simulink model "Pokus07_Display"  (Simulink 8.1)
settings: Solver=ode45  StartTime=0.0  StopTime=10.0  RelTol=1e-3
undefined symbols (not defined in the file): A, ARROW_DOWN, ARROW_LEFT, ARROW_RIGHT, ARROW_UP, ASTERISK, B, BACKSLASH, C, COLON, COMMA, CROSS, CURSOR, D, DOT, ending_column_index, ending_row_index, EQUAL, EXCLAMATION_MARK, F, framebuffer, G, GREATER_THAN, H, HEIGHT, hot, I, J, K, L, LEFT_PARENTHESES, LESS_THAN, M, MINUS, N, O, P, PERCENT, PLUS, POS_X, POS_Y, Q, QUESTION_MARK, QUOTE, R, RECTANGLE, RIGHT_PARENTHESES, S, SEMICOLON, SHARP, SLASH, SPACE, starting_column_index, starting_row_index, T, U, UNDERSCORE, V, W, WIDTH ... (+6)
libraries: dspmtrx3 x197, Common_Library x69, commutil2 x53, simulink_extras x1, dspsnks4 x1
(part 1 of 6)
settings Model: Creator=uzivatel  LastModifiedBy=uzivatel
settings DataIOCC: SignalLoggingSaveFormat=Dataset
settings OptimizationCC: ExpressionDepthLimit=128
settings DebuggingCC: FcnCallInpInsideContextMsg=EnableAllAsError
settings GRTTargetCC: CombineOutputUpdateFcns=on  GRTInterface=off

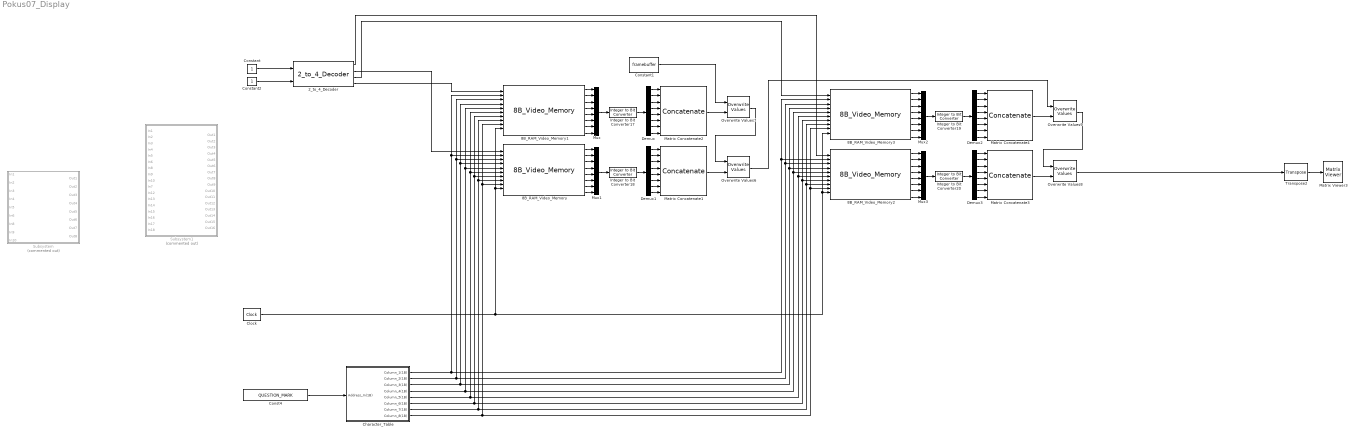
== system Pokus07_Display ==
  2_to_4_Decoder : Common_Library/Decoders/2_to_4_Decoder
  8B_RAM_Video_Memory{,1..3} (4 alike) : Common_Library/Memory_Blocks/8B_Video_Memory
  Character_Table : Subsystem
  Clock : simulink_extras/Flip Flops/Clock  period=1
  Const4 : Constant  Value=QUESTION_MARK  OutDataTypeStr=uint8
  Constant : Constant  OutDataTypeStr=boolean
  Constant1 : Constant  Value=framebuffer  OutDataTypeStr=uint8
  Constant2 : Constant  OutDataTypeStr=boolean
  Demux{,1..3} (4 alike) : Demux  Outputs=8
  Integer to Bit Converter{17..20} (4 alike) : commutil2/Integer to Bit Converter  nbits=8  signedInputValues=Unsigned  bitOrder=MSB first  outDtype=uint8
  Matrix Concatenate{1..4} (4 alike) : Concatenate  NumInputs=8  Mode=Multidimensional array  ConcatenateDimension=2
  Matrix Viewer3 : dspsnks4/Matrix Viewer  ImageParams=off  CMapStr=hot(256)  AxisColorbar=on  AxisParams=off  AxisOrigin=Upper left corner  XLabel=X-axis  YLabel=Y-axis  ZLabel=Z-axis  FigPos=[POS_X POS_Y-140 WIDTH HEIGHT]  AxisZoom=on
      settings: YMin=0  YMax=1.0
  Mux{,1..3} (4 alike) : Mux  Inputs=8
  Overwrite Values6 : dspmtrx3/Overwrite Values  OverWriteDiag=Submatrix  valFrom2ndIP=Second input port  ConstValue=0  RowSpan=Range of rows  RowStartMode=Index  RowStartIndex=starting_row_index(2)  RowEndMode=Index  RowEndIndex=ending_row_index(2)  ColSpan=Range of columns  ColStartMode=Index  ColStartIndex=starting_column_index(1)  ColEndMode=Index  ColEndIndex=ending_column_index(1)  DiagSpan=Range of elements  DiagStartMode=Index  DiagStartIndex=2  DiagEndMode=Index  DiagEndIndex=4
  Overwrite Values7 : dspmtrx3/Overwrite Values  OverWriteDiag=Submatrix  valFrom2ndIP=Second input port  ConstValue=0  RowSpan=Range of rows  RowStartMode=Index  RowStartIndex=starting_row_index(1)  RowEndMode=Index  RowEndIndex=ending_row_index(1)  ColSpan=Range of columns  ColStartMode=Index  ColStartIndex=starting_column_index(1)  ColEndMode=Index  ColEndIndex=ending_column_index(1)  DiagSpan=Range of elements  DiagStartMode=Index  DiagStartIndex=2  DiagEndMode=Index  DiagEndIndex=4
  Overwrite Values8 : dspmtrx3/Overwrite Values  OverWriteDiag=Submatrix  valFrom2ndIP=Second input port  ConstValue=0  RowSpan=Range of rows  RowStartMode=Index  RowStartIndex=starting_row_index(2)  RowEndMode=Index  RowEndIndex=ending_row_index(2)  ColSpan=Range of columns  ColStartMode=Index  ColStartIndex=starting_column_index(2)  ColEndMode=Index  ColEndIndex=ending_column_index(2)  DiagSpan=Range of elements  DiagStartMode=Index  DiagStartIndex=2  DiagEndMode=Index  DiagEndIndex=4
  Overwrite Values9 : dspmtrx3/Overwrite Values  OverWriteDiag=Submatrix  valFrom2ndIP=Second input port  ConstValue=0  RowSpan=Range of rows  RowStartMode=Index  RowStartIndex=starting_row_index(1)  RowEndMode=Index  RowEndIndex=ending_row_index(1)  ColSpan=Range of columns  ColStartMode=Index  ColStartIndex=starting_column_index(2)  ColEndMode=Index  ColEndIndex=ending_column_index(2)  DiagSpan=Range of elements  DiagStartMode=Index  DiagStartIndex=2  DiagEndMode=Index  DiagEndIndex=4
  Subsystem : Subsystem  Commented=on
  Subsystem1 : Subsystem  Commented=on
  Transpose2 : dspmtrx3/Transpose  Hermitian=off  overflowFlag=off
  wires:
  Const4/1 -> Character_Table/1(Address_In(1B))
  Matrix Concatenate1/1 -> Overwrite Values6/2
  Matrix Concatenate3/1 -> Overwrite Values8/2
  Matrix Concatenate4/1 -> Overwrite Values9/2
  Clock/1 -> 8B_RAM_Video_Memory1/10, 8B_RAM_Video_Memory/10, 8B_RAM_Video_Memory3/10, 8B_RAM_Video_Memory2/10
  Overwrite Values6/1 -> Overwrite Values9/1
  Overwrite Values9/1 -> Overwrite Values8/1
  Overwrite Values8/1 -> Transpose2/1
  2_to_4_Decoder/4 -> 8B_RAM_Video_Memory1/1
  2_to_4_Decoder/3 -> 8B_RAM_Video_Memory3/1
  2_to_4_Decoder/2 -> 8B_RAM_Video_Memory/1
  2_to_4_Decoder/1 -> 8B_RAM_Video_Memory2/1
  Character_Table/1(Column_1(1B)) -> 8B_RAM_Video_Memory2/2, 8B_RAM_Video_Memory3/2, 8B_RAM_Video_Memory1/2, 8B_RAM_Video_Memory/2
  Character_Table/2(Column_2(1B)) -> 8B_RAM_Video_Memory1/3, 8B_RAM_Video_Memory/3, 8B_RAM_Video_Memory2/3, 8B_RAM_Video_Memory3/3
  Character_Table/3(Column_3(1B)) -> 8B_RAM_Video_Memory2/4, 8B_RAM_Video_Memory3/4, 8B_RAM_Video_Memory1/4, 8B_RAM_Video_Memory/4
  Character_Table/4(Column_4(1B)) -> 8B_RAM_Video_Memory2/5, 8B_RAM_Video_Memory3/5, 8B_RAM_Video_Memory1/5, 8B_RAM_Video_Memory/5
  Character_Table/5(Column_5(1B)) -> 8B_RAM_Video_Memory2/6, 8B_RAM_Video_Memory3/6, 8B_RAM_Video_Memory1/6, 8B_RAM_Video_Memory/6
  Character_Table/6(Column_6(1B)) -> 8B_RAM_Video_Memory2/7, 8B_RAM_Video_Memory3/7, 8B_RAM_Video_Memory1/7, 8B_RAM_Video_Memory/7
  Character_Table/7(Column_7(1B)) -> 8B_RAM_Video_Memory2/8, 8B_RAM_Video_Memory3/8, 8B_RAM_Video_Memory1/8, 8B_RAM_Video_Memory/8
  Character_Table/8(Column_8(1B)) -> 8B_RAM_Video_Memory2/9, 8B_RAM_Video_Memory3/9, 8B_RAM_Video_Memory1/9, 8B_RAM_Video_Memory/9
  Constant1/1 -> Overwrite Values7/1
  Constant/1 -> 2_to_4_Decoder/1
  Constant2/1 -> 2_to_4_Decoder/2
  Matrix Concatenate2/1 -> Overwrite Values7/2
  8B_RAM_Video_Memory1/1 -> Mux/1
  8B_RAM_Video_Memory1/2 -> Mux/2
  8B_RAM_Video_Memory1/3 -> Mux/3
  8B_RAM_Video_Memory1/4 -> Mux/4
  8B_RAM_Video_Memory1/5 -> Mux/5
  8B_RAM_Video_Memory1/6 -> Mux/6
  8B_RAM_Video_Memory1/7 -> Mux/7
  8B_RAM_Video_Memory1/8 -> Mux/8
  Demux/1 -> Matrix Concatenate2/1
  Demux/2 -> Matrix Concatenate2/2
  Demux/3 -> Matrix Concatenate2/3
  Demux/4 -> Matrix Concatenate2/4
  Demux/5 -> Matrix Concatenate2/5
  Demux/6 -> Matrix Concatenate2/6
  Demux/7 -> Matrix Concatenate2/7
  Demux/8 -> Matrix Concatenate2/8
  Integer to Bit Converter17/1 -> Demux/1
  Mux/1 -> Integer to Bit Converter17/1
  8B_RAM_Video_Memory/1 -> Mux1/1
  8B_RAM_Video_Memory/2 -> Mux1/2
  8B_RAM_Video_Memory/3 -> Mux1/3
  8B_RAM_Video_Memory/4 -> Mux1/4
  8B_RAM_Video_Memory/5 -> Mux1/5
  8B_RAM_Video_Memory/6 -> Mux1/6
  8B_RAM_Video_Memory/7 -> Mux1/7
  8B_RAM_Video_Memory/8 -> Mux1/8
  Demux1/1 -> Matrix Concatenate1/1
  Demux1/2 -> Matrix Concatenate1/2
  Demux1/3 -> Matrix Concatenate1/3
  Demux1/4 -> Matrix Concatenate1/4
  Demux1/5 -> Matrix Concatenate1/5
  Demux1/6 -> Matrix Concatenate1/6
  Demux1/7 -> Matrix Concatenate1/7
  Demux1/8 -> Matrix Concatenate1/8
  Integer to Bit Converter18/1 -> Demux1/1
  Mux1/1 -> Integer to Bit Converter18/1
  8B_RAM_Video_Memory3/1 -> Mux2/1
  8B_RAM_Video_Memory3/2 -> Mux2/2
  8B_RAM_Video_Memory3/3 -> Mux2/3
  8B_RAM_Video_Memory3/4 -> Mux2/4
  8B_RAM_Video_Memory3/5 -> Mux2/5
  8B_RAM_Video_Memory3/6 -> Mux2/6
  8B_RAM_Video_Memory3/7 -> Mux2/7
  8B_RAM_Video_Memory3/8 -> Mux2/8
  Demux2/1 -> Matrix Concatenate4/1
  Demux2/2 -> Matrix Concatenate4/2
  Demux2/3 -> Matrix Concatenate4/3
  Demux2/4 -> Matrix Concatenate4/4
  Demux2/5 -> Matrix Concatenate4/5
  Demux2/6 -> Matrix Concatenate4/6
  Demux2/7 -> Matrix Concatenate4/7
  Demux2/8 -> Matrix Concatenate4/8
  Integer to Bit Converter19/1 -> Demux2/1
  Mux2/1 -> Integer to Bit Converter19/1
  8B_RAM_Video_Memory2/1 -> Mux3/1
  8B_RAM_Video_Memory2/2 -> Mux3/2
  8B_RAM_Video_Memory2/3 -> Mux3/3
  8B_RAM_Video_Memory2/4 -> Mux3/4
  8B_RAM_Video_Memory2/5 -> Mux3/5
  8B_RAM_Video_Memory2/6 -> Mux3/6
  8B_RAM_Video_Memory2/7 -> Mux3/7
  8B_RAM_Video_Memory2/8 -> Mux3/8
  Demux3/1 -> Matrix Concatenate3/1
  Demux3/2 -> Matrix Concatenate3/2
  Demux3/3 -> Matrix Concatenate3/3
  Demux3/4 -> Matrix Concatenate3/4
  Demux3/5 -> Matrix Concatenate3/5
  Demux3/6 -> Matrix Concatenate3/6
  Demux3/7 -> Matrix Concatenate3/7
  Demux3/8 -> Matrix Concatenate3/8
  Integer to Bit Converter20/1 -> Demux3/1
  Mux3/1 -> Integer to Bit Converter20/1
  Transpose2/1 -> Matrix Viewer3/1
  Overwrite Values7/1 -> Overwrite Values6/1

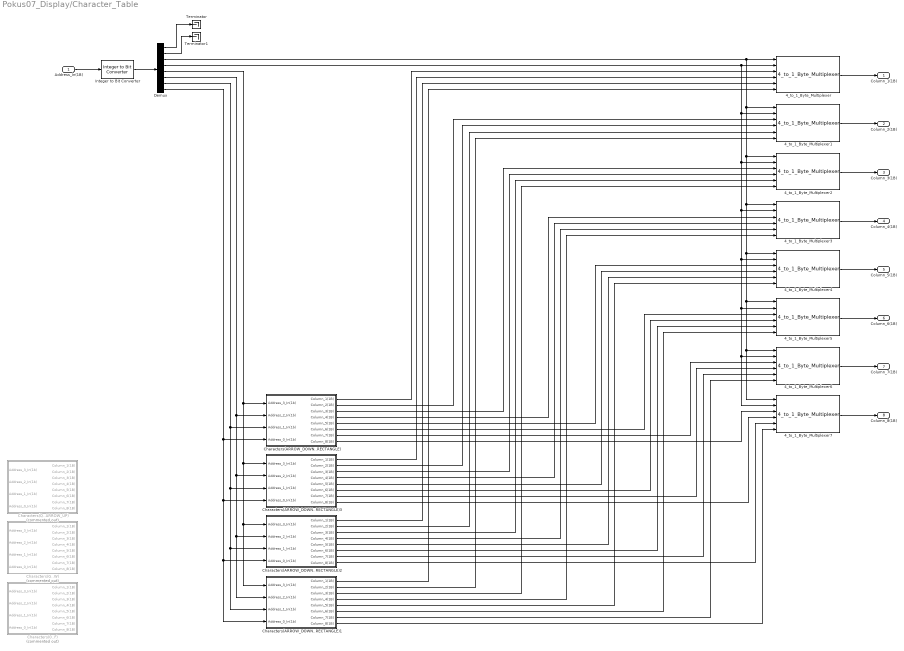
== system Pokus07_Display/Character_Table ==
  Address_In(1B) : Inport
  4_to_1_Byte_Multiplexer{,1..7} (8 alike) : Common_Library/Multiplexers/4_to_1_Byte_Multiplexer
  Characters(0..F) : Subsystem  Commented=on
  Characters(ARROW_DOWN..RECTANGLE) : Subsystem
  Characters(ARROW_DOWN..RECTANGLE)1 : Subsystem
  Characters(ARROW_DOWN..RECTANGLE)2 : Subsystem
  Characters(ARROW_DOWN..RECTANGLE)3 : Subsystem
  Characters(G..W) : Subsystem  Commented=on
  Characters(Q..ARROW_UP) : Subsystem  Commented=on
  Demux : Demux  Outputs=8
  Integer to Bit Converter : commutil2/Integer to Bit Converter  nbits=8  signedInputValues=Unsigned  bitOrder=MSB first  outDtype=uint8
  Terminator : Terminator
  Terminator1 : Terminator
  Column_1(1B) : Outport
  Column_2(1B) : Outport  Port=2
  Column_3(1B) : Outport  Port=3
  Column_4(1B) : Outport  Port=4
  Column_5(1B) : Outport  Port=5
  Column_6(1B) : Outport  Port=6
  Column_7(1B) : Outport  Port=7
  Column_8(1B) : Outport  Port=8
  wires:
  Characters(ARROW_DOWN..RECTANGLE)1/3(Column_3(1B)) -> 4_to_1_Byte_Multiplexer2/6
  Characters(ARROW_DOWN..RECTANGLE)3/6(Column_6(1B)) -> 4_to_1_Byte_Multiplexer5/4
  Characters(ARROW_DOWN..RECTANGLE)3/7(Column_7(1B)) -> 4_to_1_Byte_Multiplexer6/4
  Characters(ARROW_DOWN..RECTANGLE)/2(Column_2(1B)) -> 4_to_1_Byte_Multiplexer1/3
  Characters(ARROW_DOWN..RECTANGLE)1/2(Column_2(1B)) -> 4_to_1_Byte_Multiplexer1/6
  Characters(ARROW_DOWN..RECTANGLE)3/2(Column_2(1B)) -> 4_to_1_Byte_Multiplexer1/4
  Characters(ARROW_DOWN..RECTANGLE)/7(Column_7(1B)) -> 4_to_1_Byte_Multiplexer6/3
  Characters(ARROW_DOWN..RECTANGLE)2/2(Column_2(1B)) -> 4_to_1_Byte_Multiplexer1/5
  Characters(ARROW_DOWN..RECTANGLE)/8(Column_8(1B)) -> 4_to_1_Byte_Multiplexer7/3
  Characters(ARROW_DOWN..RECTANGLE)2/4(Column_4(1B)) -> 4_to_1_Byte_Multiplexer3/5
  Characters(ARROW_DOWN..RECTANGLE)/6(Column_6(1B)) -> 4_to_1_Byte_Multiplexer5/3
  Characters(ARROW_DOWN..RECTANGLE)2/3(Column_3(1B)) -> 4_to_1_Byte_Multiplexer2/5
  Characters(ARROW_DOWN..RECTANGLE)3/5(Column_5(1B)) -> 4_to_1_Byte_Multiplexer4/4
  Characters(ARROW_DOWN..RECTANGLE)1/4(Column_4(1B)) -> 4_to_1_Byte_Multiplexer3/6
  Characters(ARROW_DOWN..RECTANGLE)3/1(Column_1(1B)) -> 4_to_1_Byte_Multiplexer/4
  Characters(ARROW_DOWN..RECTANGLE)/3(Column_3(1B)) -> 4_to_1_Byte_Multiplexer2/3
  Characters(ARROW_DOWN..RECTANGLE)3/3(Column_3(1B)) -> 4_to_1_Byte_Multiplexer2/4
  Characters(ARROW_DOWN..RECTANGLE)2/6(Column_6(1B)) -> 4_to_1_Byte_Multiplexer5/5
  Characters(ARROW_DOWN..RECTANGLE)1/7(Column_7(1B)) -> 4_to_1_Byte_Multiplexer6/6
  Characters(ARROW_DOWN..RECTANGLE)2/7(Column_7(1B)) -> 4_to_1_Byte_Multiplexer6/5
  Characters(ARROW_DOWN..RECTANGLE)1/8(Column_8(1B)) -> 4_to_1_Byte_Multiplexer7/6
  Characters(ARROW_DOWN..RECTANGLE)3/8(Column_8(1B)) -> 4_to_1_Byte_Multiplexer7/4
  Characters(ARROW_DOWN..RECTANGLE)/5(Column_5(1B)) -> 4_to_1_Byte_Multiplexer4/3
  Characters(ARROW_DOWN..RECTANGLE)2/8(Column_8(1B)) -> 4_to_1_Byte_Multiplexer7/5
  Demux/3 -> 4_to_1_Byte_Multiplexer1/1, 4_to_1_Byte_Multiplexer2/1, 4_to_1_Byte_Multiplexer4/1, 4_to_1_Byte_Multiplexer5/1, 4_to_1_Byte_Multiplexer6/1, 4_to_1_Byte_Multiplexer7/1, 4_to_1_Byte_Multiplexer3/1, 4_to_1_Byte_Multiplexer/1
  Characters(ARROW_DOWN..RECTANGLE)3/4(Column_4(1B)) -> 4_to_1_Byte_Multiplexer3/4
  Demux/4 -> 4_to_1_Byte_Multiplexer1/2, 4_to_1_Byte_Multiplexer2/2, 4_to_1_Byte_Multiplexer3/2, 4_to_1_Byte_Multiplexer4/2, 4_to_1_Byte_Multiplexer5/2, 4_to_1_Byte_Multiplexer6/2, 4_to_1_Byte_Multiplexer7/2, 4_to_1_Byte_Multiplexer/2
  Characters(ARROW_DOWN..RECTANGLE)1/1(Column_1(1B)) -> 4_to_1_Byte_Multiplexer/6
  Characters(ARROW_DOWN..RECTANGLE)2/1(Column_1(1B)) -> 4_to_1_Byte_Multiplexer/5
  Characters(ARROW_DOWN..RECTANGLE)1/5(Column_5(1B)) -> 4_to_1_Byte_Multiplexer4/6
  Characters(ARROW_DOWN..RECTANGLE)2/5(Column_5(1B)) -> 4_to_1_Byte_Multiplexer4/5
  Characters(ARROW_DOWN..RECTANGLE)1/6(Column_6(1B)) -> 4_to_1_Byte_Multiplexer5/6
  Characters(ARROW_DOWN..RECTANGLE)/1(Column_1(1B)) -> 4_to_1_Byte_Multiplexer/3
  Characters(ARROW_DOWN..RECTANGLE)/4(Column_4(1B)) -> 4_to_1_Byte_Multiplexer3/3
  Demux/8 -> Characters(ARROW_DOWN..RECTANGLE)/4(Address_0_In(1b)), Characters(ARROW_DOWN..RECTANGLE)3/4(Address_0_In(1b)), Characters(ARROW_DOWN..RECTANGLE)1/4(Address_0_In(1b)), Characters(ARROW_DOWN..RECTANGLE)2/4(Address_0_In(1b))
  Demux/6 -> Characters(ARROW_DOWN..RECTANGLE)/2(Address_2_In(1b)), Characters(ARROW_DOWN..RECTANGLE)3/2(Address_2_In(1b)), Characters(ARROW_DOWN..RECTANGLE)1/2(Address_2_In(1b)), Characters(ARROW_DOWN..RECTANGLE)2/2(Address_2_In(1b))
  4_to_1_Byte_Multiplexer6/1 -> Column_7(1B)/1
  Demux/5 -> Characters(ARROW_DOWN..RECTANGLE)/1(Address_3_In(1b)), Characters(ARROW_DOWN..RECTANGLE)3/1(Address_3_In(1b)), Characters(ARROW_DOWN..RECTANGLE)1/1(Address_3_In(1b)), Characters(ARROW_DOWN..RECTANGLE)2/1(Address_3_In(1b))
  4_to_1_Byte_Multiplexer1/1 -> Column_2(1B)/1
  4_to_1_Byte_Multiplexer5/1 -> Column_6(1B)/1
  4_to_1_Byte_Multiplexer2/1 -> Column_3(1B)/1
  4_to_1_Byte_Multiplexer3/1 -> Column_4(1B)/1
  4_to_1_Byte_Multiplexer7/1 -> Column_8(1B)/1
  4_to_1_Byte_Multiplexer/1 -> Column_1(1B)/1
  Demux/7 -> Characters(ARROW_DOWN..RECTANGLE)/3(Address_1_In(1b)), Characters(ARROW_DOWN..RECTANGLE)3/3(Address_1_In(1b)), Characters(ARROW_DOWN..RECTANGLE)1/3(Address_1_In(1b)), Characters(ARROW_DOWN..RECTANGLE)2/3(Address_1_In(1b))
  4_to_1_Byte_Multiplexer4/1 -> Column_5(1B)/1
  Address_In(1B)/1 -> Integer to Bit Converter/1
  Demux/1 -> Terminator/1
  Demux/2 -> Terminator1/1
  Integer to Bit Converter/1 -> Demux/1

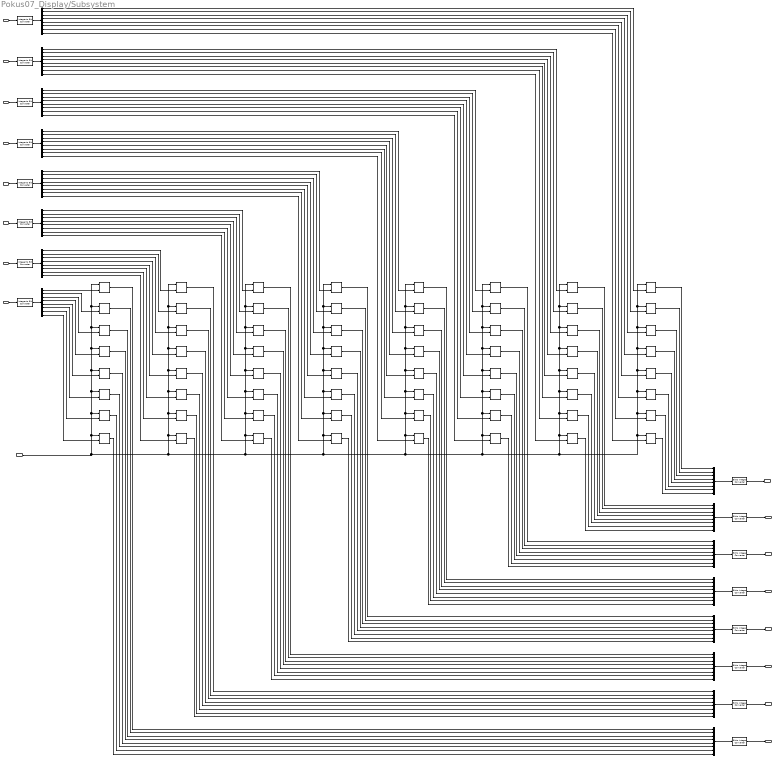
== system Pokus07_Display/Subsystem ==
  In1 : Inport
  In2 : Inport  Port=2
  In3 : Inport  Port=3
  In4 : Inport  Port=4
  In5 : Inport  Port=5
  In6 : Inport  Port=6
  In8 : Inport  Port=7
  In9 : Inport  Port=8
  In10 : Inport  Port=9
  Bit to Integer Converter{,1..7} (8 alike) : commutil2/Bit to Integer Converter  nbits=8  bitOrder=MSB first  signedOutputValues=Unsigned  outDtype=uint8  outDtypeSigned=Inherit via internal rule
  Demux{,1..7} (8 alike) : Demux  Outputs=8
  Integer to Bit Converter{,1..7} (8 alike) : commutil2/Integer to Bit Converter  nbits=8  signedInputValues=Signed  bitOrder=MSB first  outDtype=uint8
  Mux{,1..7} (8 alike) : Mux  Inputs=8
  Overwrite Values{5..10,12..67} (62 alike) : dspmtrx3/Overwrite Values  OverWriteDiag=Submatrix  valFrom2ndIP=Second input port  ConstValue=0  RowSpan=One row  RowStartMode=Index  RowStartIndex=1  RowEndMode=Index  RowEndIndex=8  ColSpan=One column  ColStartMode=Index  ColStartIndex=1  ColEndMode=Index  ColEndIndex=8  DiagSpan=Range of elements  DiagStartMode=Index  DiagStartIndex=2  DiagEndMode=Index  DiagEndIndex=4
  Overwrite Values11 : dspmtrx3/Overwrite Values  OverWriteDiag=Submatrix  valFrom2ndIP=Second input port  ConstValue=0  RowSpan=One row  RowStartMode=Index  RowStartIndex=Y_OFFSET + 0  RowEndMode=Index  RowEndIndex=8  ColSpan=One column  ColStartMode=Index  ColStartIndex=X_OFFSET + 0  ColEndMode=Index  ColEndIndex=8  DiagSpan=Range of elements  DiagStartMode=Index  DiagStartIndex=2  DiagEndMode=Index  DiagEndIndex=4
  Overwrite Values4 : dspmtrx3/Overwrite Values  OverWriteDiag=Submatrix  valFrom2ndIP=Second input port  ConstValue=0  RowSpan=One row  RowStartMode=Index  RowStartIndex=Y_OFFSET + 1  RowEndMode=Index  RowEndIndex=8  ColSpan=One column  ColStartMode=Index  ColStartIndex=X_OFFSET + 0  ColEndMode=Index  ColEndIndex=8  DiagSpan=Range of elements  DiagStartMode=Index  DiagStartIndex=2  DiagEndMode=Index  DiagEndIndex=4
  Out1 : Outport
  Out2 : Outport  Port=2
  Out3 : Outport  Port=3
  Out4 : Outport  Port=4
  Out5 : Outport  Port=5
  Out6 : Outport  Port=6
  Out7 : Outport  Port=7
  Out8 : Outport  Port=8
  wires:
  Bit to Integer Converter/1 -> Out1/1
  Mux/1 -> Bit to Integer Converter/1
  Demux/1 -> Overwrite Values11/2
  Overwrite Values26/1 -> Mux2/6
  Overwrite Values20/1 -> Mux2/8
  Overwrite Values27/1 -> Mux2/7
  Mux5/1 -> Bit to Integer Converter5/1
  Demux3/6 -> Overwrite Values34/2
  Overwrite Values31/1 -> Mux3/3
  Overwrite Values39/1 -> Mux5/1
  Demux7/1 -> Overwrite Values55/2
  Integer to Bit Converter7/1 -> Demux7/1
  Mux3/1 -> Bit to Integer Converter3/1
  Overwrite Values29/1 -> Mux3/1
  Overwrite Values28/1 -> Mux3/8
  Demux3/5 -> Overwrite Values33/2
  Demux5/8 -> Overwrite Values38/2
  Demux3/7 -> Overwrite Values35/2
  Overwrite Values33/1 -> Mux3/5
  Demux3/8 -> Overwrite Values28/2
  In5/1 -> Integer to Bit Converter3/1
  Demux3/1 -> Overwrite Values29/2
  Demux3/4 -> Overwrite Values32/2
  Integer to Bit Converter3/1 -> Demux3/1
  Overwrite Values34/1 -> Mux3/6
  Demux3/2 -> Overwrite Values30/2
  Overwrite Values60/1 -> Mux7/6
  Overwrite Values40/1 -> Mux5/2
  Overwrite Values30/1 -> Mux3/2
  Bit to Integer Converter3/1 -> Out4/1
  Overwrite Values32/1 -> Mux3/4
  Demux4/3 -> Overwrite Values63/2
  Overwrite Values61/1 -> Mux7/7
  Overwrite Values49/1 -> Mux6/3
  Overwrite Values58/1 -> Mux7/4
  Demux5/3 -> Overwrite Values41/2
  Overwrite Values48/1 -> Mux6/2
  Overwrite Values52/1 -> Mux6/6
  Demux6/4 -> Overwrite Values50/2
  Demux7/2 -> Overwrite Values56/2
  Demux6/3 -> Overwrite Values49/2
  Demux6/6 -> Overwrite Values52/2
  Demux7/3 -> Overwrite Values57/2
  Demux4/2 -> Overwrite Values62/2
  Overwrite Values37/1 -> Mux4/1
  Overwrite Values59/1 -> Mux7/5
  Overwrite Values44/1 -> Mux5/6
  Overwrite Values36/1 -> Mux4/8
  In2/1 -> Overwrite Values11/1, Overwrite Values4/1, Overwrite Values5/1, Overwrite Values6/1, Overwrite Values7/1, Overwrite Values8/1, Overwrite Values9/1, Overwrite Values10/1, Overwrite Values37/1, Overwrite Values62/1, Overwrite Values63/1, Overwrite Values64/1, Overwrite Values65/1, Overwrite Values66/1, Overwrite Values67/1, Overwrite Values36/1, Overwrite Values55/1, Overwrite Values56/1, Overwrite Values57/1, Overwrite Values58/1, Overwrite Values59/1, Overwrite Values60/1, Overwrite Values61/1, Overwrite Values54/1, Overwrite Values47/1, Overwrite Values48/1, Overwrite Values49/1, Overwrite Values50/1, Overwrite Values51/1, Overwrite Values52/1, Overwrite Values53/1, Overwrite Values46/1, Overwrite Values39/1, Overwrite Values40/1, Overwrite Values41/1, Overwrite Values42/1, Overwrite Values43/1, Overwrite Values44/1, Overwrite Values45/1, Overwrite Values38/1, Overwrite Values29/1, Overwrite Values30/1, Overwrite Values31/1, Overwrite Values32/1, Overwrite Values33/1, Overwrite Values34/1, Overwrite Values35/1, Overwrite Values28/1, Overwrite Values21/1, Overwrite Values22/1, Overwrite Values23/1, Overwrite Values24/1, Overwrite Values25/1, Overwrite Values26/1, Overwrite Values27/1, Overwrite Values20/1, Overwrite Values13/1, Overwrite Values14/1, Overwrite Values15/1, Overwrite Values16/1, Overwrite Values17/1, Overwrite Values18/1, Overwrite Values19/1, Overwrite Values12/1
  Mux7/1 -> Bit to Integer Converter7/1
  Overwrite Values62/1 -> Mux4/2
  Overwrite Values38/1 -> Mux5/8
  Overwrite Values54/1 -> Mux7/8
  In10/1 -> Integer to Bit Converter7/1
  Demux6/5 -> Overwrite Values51/2
  Demux5/1 -> Overwrite Values39/2
  Overwrite Values47/1 -> Mux6/1
  Demux4/8 -> Overwrite Values36/2
  Overwrite Values67/1 -> Mux4/7
  Demux7/4 -> Overwrite Values58/2
  Demux6/7 -> Overwrite Values53/2
  Demux5/2 -> Overwrite Values40/2
  Bit to Integer Converter6/1 -> Out7/1
  Overwrite Values45/1 -> Mux5/7
  Demux6/2 -> Overwrite Values48/2
  Demux6/1 -> Overwrite Values47/2
  Integer to Bit Converter6/1 -> Demux6/1
  In9/1 -> Integer to Bit Converter6/1
  Demux7/5 -> Overwrite Values59/2
  Overwrite Values57/1 -> Mux7/3
  Demux7/6 -> Overwrite Values60/2
  Demux7/7 -> Overwrite Values61/2
  Demux7/8 -> Overwrite Values54/2
  Mux4/1 -> Bit to Integer Converter4/1
  Overwrite Values56/1 -> Mux7/2
  Demux6/8 -> Overwrite Values46/2
  Mux6/1 -> Bit to Integer Converter6/1
  In6/1 -> Integer to Bit Converter4/1
  Overwrite Values51/1 -> Mux6/5
  Overwrite Values53/1 -> Mux6/7
  Overwrite Values50/1 -> Mux6/4
  Bit to Integer Converter7/1 -> Out8/1
  Overwrite Values66/1 -> Mux4/6
  Overwrite Values65/1 -> Mux4/5
  Overwrite Values64/1 -> Mux4/4
  Overwrite Values63/1 -> Mux4/3
  Bit to Integer Converter4/1 -> Out5/1
  Overwrite Values55/1 -> Mux7/1
  Demux4/7 -> Overwrite Values67/2
  Demux4/4 -> Overwrite Values64/2
  Demux4/6 -> Overwrite Values66/2
  Demux4/5 -> Overwrite Values65/2
  In8/1 -> Integer to Bit Converter5/1
  Integer to Bit Converter5/1 -> Demux5/1
  Demux4/1 -> Overwrite Values37/2
  Demux5/4 -> Overwrite Values42/2
  Demux5/5 -> Overwrite Values43/2
  Demux5/6 -> Overwrite Values44/2
  Demux5/7 -> Overwrite Values45/2
  Integer to Bit Converter4/1 -> Demux4/1
  Overwrite Values41/1 -> Mux5/3
  Bit to Integer Converter5/1 -> Out6/1
  Overwrite Values42/1 -> Mux5/4
  Overwrite Values46/1 -> Mux6/8
  Overwrite Values43/1 -> Mux5/5
  Demux3/3 -> Overwrite Values31/2
  Overwrite Values35/1 -> Mux3/7
  In4/1 -> Integer to Bit Converter2/1
  Demux1/1 -> Overwrite Values13/2
  Overwrite Values14/1 -> Mux1/2
  Overwrite Values18/1 -> Mux1/6
  Bit to Integer Converter2/1 -> Out3/1
  Demux2/1 -> Overwrite Values21/2
  Integer to Bit Converter1/1 -> Demux1/1
  Demux1/2 -> Overwrite Values14/2
  Demux2/6 -> Overwrite Values26/2
  Demux/5 -> Overwrite Values7/2
  Overwrite Values6/1 -> Mux/4
  Demux/3 -> Overwrite Values5/2
  Demux1/8 -> Overwrite Values12/2
  Overwrite Values8/1 -> Mux/6
  Demux/7 -> Overwrite Values9/2
  Overwrite Values11/1 -> Mux/1
  Demux/6 -> Overwrite Values8/2
  Overwrite Values17/1 -> Mux1/5
  Demux/4 -> Overwrite Values6/2
  In3/1 -> Integer to Bit Converter1/1
  Overwrite Values15/1 -> Mux1/3
  Demux/2 -> Overwrite Values4/2
  Demux2/8 -> Overwrite Values20/2
  Overwrite Values21/1 -> Mux2/1
  Demux1/5 -> Overwrite Values17/2
  Overwrite Values23/1 -> Mux2/3
  Demux2/7 -> Overwrite Values27/2
  In1/1 -> Integer to Bit Converter/1
  Demux1/4 -> Overwrite Values16/2
  Integer to Bit Converter/1 -> Demux/1
  Demux2/2 -> Overwrite Values22/2
  Demux/8 -> Overwrite Values10/2
  Overwrite Values10/1 -> Mux/8
  Demux1/7 -> Overwrite Values19/2
  Overwrite Values25/1 -> Mux2/5
  Overwrite Values5/1 -> Mux/3
  Demux1/6 -> Overwrite Values18/2
  Overwrite Values19/1 -> Mux1/7
  Mux1/1 -> Bit to Integer Converter1/1
  Overwrite Values9/1 -> Mux/7
  Overwrite Values24/1 -> Mux2/4
  Mux2/1 -> Bit to Integer Converter2/1
  Overwrite Values16/1 -> Mux1/4
  Overwrite Values22/1 -> Mux2/2
  Demux2/3 -> Overwrite Values23/2
  Overwrite Values7/1 -> Mux/5
  Demux1/3 -> Overwrite Values15/2
  Demux2/5 -> Overwrite Values25/2
  Overwrite Values12/1 -> Mux1/8
  Integer to Bit Converter2/1 -> Demux2/1
  Overwrite Values13/1 -> Mux1/1
  Overwrite Values4/1 -> Mux/2
  Bit to Integer Converter1/1 -> Out2/1
  Demux2/4 -> Overwrite Values24/2

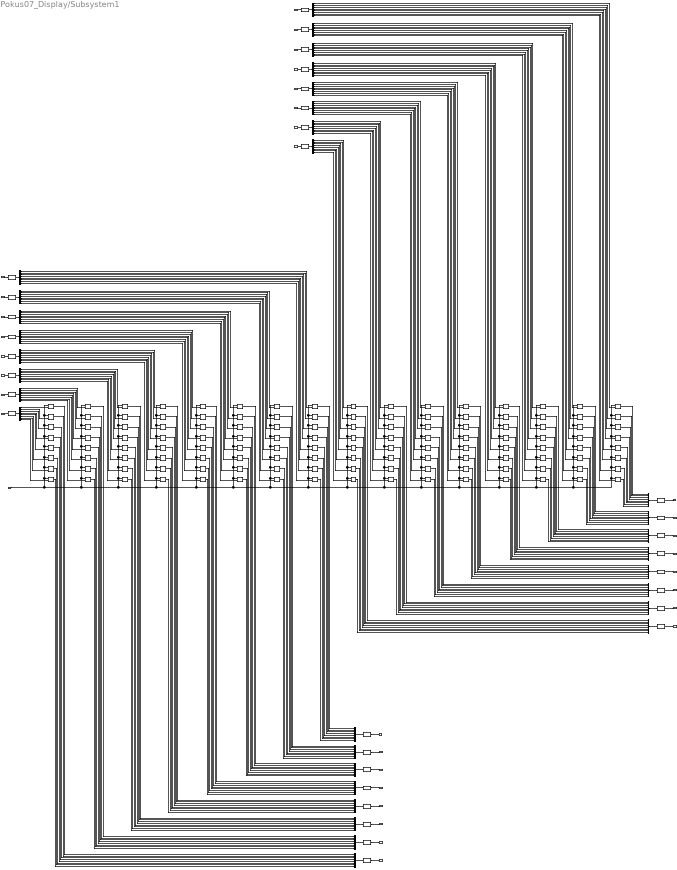
== system Pokus07_Display/Subsystem1 ==
  In1 : Inport
  In2 : Inport  Port=2
  In3 : Inport  Port=3
  In4 : Inport  Port=4
  In5 : Inport  Port=5
  In6 : Inport  Port=6
  In8 : Inport  Port=7
  In9 : Inport  Port=8
  In10 : Inport  Port=9
  In7 : Inport  Port=10
  In12 : Inport  Port=11
  In13 : Inport  Port=12
  In14 : Inport  Port=13
  In15 : Inport  Port=14
  In16 : Inport  Port=15
  In17 : Inport  Port=16
  In18 : Inport  Port=17
  Bit to Integer Converter{,1..15} (16 alike) : commutil2/Bit to Integer Converter  nbits=8  bitOrder=MSB first  signedOutputValues=Unsigned  outDtype=uint8  outDtypeSigned=Inherit via internal rule
  Demux{,1..15} (16 alike) : Demux  Outputs=8
  Integer to Bit Converter{,1..15} (16 alike) : commutil2/Integer to Bit Converter  nbits=8  signedInputValues=Signed  bitOrder=MSB first  outDtype=uint8
  Mux{,1..15} (16 alike) : Mux  Inputs=8
  Overwrite Values{1,3,5..10,12..94,96..128} (124 alike) : dspmtrx3/Overwrite Values  OverWriteDiag=Submatrix  valFrom2ndIP=Second input port  ConstValue=0  RowSpan=One row  RowStartMode=Index  RowStartIndex=1  RowEndMode=Index  RowEndIndex=8  ColSpan=One column  ColStartMode=Index  ColStartIndex=1  ColEndMode=Index  ColEndIndex=8  DiagSpan=Range of elements  DiagStartMode=Index  DiagStartIndex=2  DiagEndMode=Index  DiagEndIndex=4
  Overwrite Values11 : dspmtrx3/Overwrite Values  OverWriteDiag=Submatrix  valFrom2ndIP=Second input port  ConstValue=0  RowSpan=One row  RowStartMode=Index  RowStartIndex=Y_OFFSET + 0  RowEndMode=Index  RowEndIndex=8  ColSpan=One column  ColStartMode=Index  ColStartIndex=X_OFFSET + 0  ColEndMode=Index  ColEndIndex=8  DiagSpan=Range of elements  DiagStartMode=Index  DiagStartIndex=2  DiagEndMode=Index  DiagEndIndex=4
  Overwrite Values2 : dspmtrx3/Overwrite Values  OverWriteDiag=Submatrix  valFrom2ndIP=Second input port  ConstValue=0  RowSpan=One row  RowStartMode=Index  RowStartIndex=Y_OFFSET + 0  RowEndMode=Index  RowEndIndex=8  ColSpan=One column  ColStartMode=Index  ColStartIndex=X_OFFSET + 0  ColEndMode=Index  ColEndIndex=8  DiagSpan=Range of elements  DiagStartMode=Index  DiagStartIndex=2  DiagEndMode=Index  DiagEndIndex=4
  Overwrite Values4 : dspmtrx3/Overwrite Values  OverWriteDiag=Submatrix  valFrom2ndIP=Second input port  ConstValue=0  RowSpan=One row  RowStartMode=Index  RowStartIndex=Y_OFFSET + 1  RowEndMode=Index  RowEndIndex=8  ColSpan=One column  ColStartMode=Index  ColStartIndex=X_OFFSET + 0  ColEndMode=Index  ColEndIndex=8  DiagSpan=Range of elements  DiagStartMode=Index  DiagStartIndex=2  DiagEndMode=Index  DiagEndIndex=4
  Overwrite Values95 : dspmtrx3/Overwrite Values  OverWriteDiag=Submatrix  valFrom2ndIP=Second input port  ConstValue=0  RowSpan=One row  RowStartMode=Index  RowStartIndex=Y_OFFSET + 1  RowEndMode=Index  RowEndIndex=8  ColSpan=One column  ColStartMode=Index  ColStartIndex=X_OFFSET + 0  ColEndMode=Index  ColEndIndex=8  DiagSpan=Range of elements  DiagStartMode=Index  DiagStartIndex=2  DiagEndMode=Index  DiagEndIndex=4
  Out1 : Outport
  Out2 : Outport  Port=2
  Out3 : Outport  Port=3
  Out4 : Outport  Port=4
  Out5 : Outport  Port=5
  Out6 : Outport  Port=6
  Out7 : Outport  Port=7
  Out8 : Outport  Port=8
  Out9 : Outport  Port=9
  Out10 : Outport  Port=10
  Out11 : Outport  Port=11
  Out12 : Outport  Port=12
  Out13 : Outport  Port=13
  Out14 : Outport  Port=14
  Out15 : Outport  Port=15
  Out16 : Outport  Port=16
  wires:
  Bit to Integer Converter/1 -> Out1/1
  Mux/1 -> Bit to Integer Converter/1
  Demux/1 -> Overwrite Values11/2
  Overwrite Values26/1 -> Mux2/6
  Overwrite Values20/1 -> Mux2/8
  Overwrite Values27/1 -> Mux2/7
  Mux5/1 -> Bit to Integer Converter5/1
  Demux3/6 -> Overwrite Values34/2
  Overwrite Values31/1 -> Mux3/3
  Overwrite Values39/1 -> Mux5/1
  Demux7/1 -> Overwrite Values55/2
  Integer to Bit Converter7/1 -> Demux7/1
  Mux3/1 -> Bit to Integer Converter3/1
  Overwrite Values29/1 -> Mux3/1
  Overwrite Values28/1 -> Mux3/8
  Demux3/5 -> Overwrite Values33/2
  Demux5/8 -> Overwrite Values38/2
  Demux3/7 -> Overwrite Values35/2
  Overwrite Values33/1 -> Mux3/5
  Demux3/8 -> Overwrite Values28/2
  In5/1 -> Integer to Bit Converter3/1
  Demux3/1 -> Overwrite Values29/2
  Demux3/4 -> Overwrite Values32/2
  Integer to Bit Converter3/1 -> Demux3/1
  Overwrite Values34/1 -> Mux3/6
  Demux3/2 -> Overwrite Values30/2
  Overwrite Values60/1 -> Mux7/6
  Overwrite Values40/1 -> Mux5/2
  Overwrite Values30/1 -> Mux3/2
  Bit to Integer Converter3/1 -> Out4/1
  Overwrite Values32/1 -> Mux3/4
  Demux4/3 -> Overwrite Values63/2
  Overwrite Values61/1 -> Mux7/7
  Overwrite Values49/1 -> Mux6/3
  Overwrite Values58/1 -> Mux7/4
  Demux5/3 -> Overwrite Values41/2
  Overwrite Values48/1 -> Mux6/2
  Overwrite Values52/1 -> Mux6/6
  Demux6/4 -> Overwrite Values50/2
  Demux7/2 -> Overwrite Values56/2
  Demux6/3 -> Overwrite Values49/2
  Demux6/6 -> Overwrite Values52/2
  Demux7/3 -> Overwrite Values57/2
  Demux4/2 -> Overwrite Values62/2
  Overwrite Values37/1 -> Mux4/1
  Overwrite Values59/1 -> Mux7/5
  Overwrite Values44/1 -> Mux5/6
  Overwrite Values36/1 -> Mux4/8
  Mux7/1 -> Bit to Integer Converter7/1
  Overwrite Values62/1 -> Mux4/2
  Overwrite Values38/1 -> Mux5/8
  Overwrite Values54/1 -> Mux7/8
  In10/1 -> Integer to Bit Converter7/1
  Demux6/5 -> Overwrite Values51/2
  Demux5/1 -> Overwrite Values39/2
  Overwrite Values47/1 -> Mux6/1
  Demux4/8 -> Overwrite Values36/2
  Overwrite Values67/1 -> Mux4/7
  Demux7/4 -> Overwrite Values58/2
  Demux6/7 -> Overwrite Values53/2
  Demux5/2 -> Overwrite Values40/2
  Bit to Integer Converter6/1 -> Out7/1
  Overwrite Values45/1 -> Mux5/7
  Demux6/2 -> Overwrite Values48/2
  Demux6/1 -> Overwrite Values47/2
  Integer to Bit Converter6/1 -> Demux6/1
  In9/1 -> Integer to Bit Converter6/1
  Demux7/5 -> Overwrite Values59/2
  Overwrite Values57/1 -> Mux7/3
  Demux7/6 -> Overwrite Values60/2
  Demux7/7 -> Overwrite Values61/2
  Demux7/8 -> Overwrite Values54/2
  Mux4/1 -> Bit to Integer Converter4/1
  Overwrite Values56/1 -> Mux7/2
  Demux6/8 -> Overwrite Values46/2
  Mux6/1 -> Bit to Integer Converter6/1
  In6/1 -> Integer to Bit Converter4/1
  Overwrite Values51/1 -> Mux6/5
  Overwrite Values53/1 -> Mux6/7
  Overwrite Values50/1 -> Mux6/4
  Bit to Integer Converter7/1 -> Out8/1
  Overwrite Values66/1 -> Mux4/6
  Overwrite Values65/1 -> Mux4/5
  Overwrite Values64/1 -> Mux4/4
  Overwrite Values63/1 -> Mux4/3
  Bit to Integer Converter4/1 -> Out5/1
  Overwrite Values55/1 -> Mux7/1
  Demux4/7 -> Overwrite Values67/2
  Demux4/4 -> Overwrite Values64/2
  Demux4/6 -> Overwrite Values66/2
  Demux4/5 -> Overwrite Values65/2
  In8/1 -> Integer to Bit Converter5/1
  Integer to Bit Converter5/1 -> Demux5/1
  Demux4/1 -> Overwrite Values37/2
  Demux5/4 -> Overwrite Values42/2
  Demux5/5 -> Overwrite Values43/2
  Demux5/6 -> Overwrite Values44/2
  Demux5/7 -> Overwrite Values45/2
  Integer to Bit Converter4/1 -> Demux4/1
  Overwrite Values41/1 -> Mux5/3
  Bit to Integer Converter5/1 -> Out6/1
  Overwrite Values42/1 -> Mux5/4
  Overwrite Values46/1 -> Mux6/8
  Overwrite Values43/1 -> Mux5/5
  Demux3/3 -> Overwrite Values31/2
  Overwrite Values35/1 -> Mux3/7
  In4/1 -> Integer to Bit Converter2/1
  Demux1/1 -> Overwrite Values13/2
  Overwrite Values14/1 -> Mux1/2
  Overwrite Values18/1 -> Mux1/6
  Bit to Integer Converter2/1 -> Out3/1
  Demux2/1 -> Overwrite Values21/2
  Integer to Bit Converter1/1 -> Demux1/1
  Demux1/2 -> Overwrite Values14/2
  Demux2/6 -> Overwrite Values26/2
  Demux/5 -> Overwrite Values7/2
  Overwrite Values6/1 -> Mux/4
  Demux/3 -> Overwrite Values5/2
  Demux1/8 -> Overwrite Values12/2
  Overwrite Values8/1 -> Mux/6
  Demux/7 -> Overwrite Values9/2
  Overwrite Values11/1 -> Mux/1
  Demux/6 -> Overwrite Values8/2
  Overwrite Values17/1 -> Mux1/5
  Demux/4 -> Overwrite Values6/2
  In3/1 -> Integer to Bit Converter1/1
  Overwrite Values15/1 -> Mux1/3
  Demux/2 -> Overwrite Values4/2
  Demux2/8 -> Overwrite Values20/2
  Overwrite Values21/1 -> Mux2/1
  Demux1/5 -> Overwrite Values17/2
  Overwrite Values23/1 -> Mux2/3
  Demux2/7 -> Overwrite Values27/2
  In1/1 -> Integer to Bit Converter/1
  Demux1/4 -> Overwrite Values16/2
  Integer to Bit Converter/1 -> Demux/1
  Demux2/2 -> Overwrite Values22/2
  Demux/8 -> Overwrite Values10/2
  Overwrite Values10/1 -> Mux/8
  Demux1/7 -> Overwrite Values19/2
  Overwrite Values25/1 -> Mux2/5
  Overwrite Values5/1 -> Mux/3
  Demux1/6 -> Overwrite Values18/2
  Overwrite Values19/1 -> Mux1/7
  Mux1/1 -> Bit to Integer Converter1/1
  Overwrite Values9/1 -> Mux/7
  Overwrite Values24/1 -> Mux2/4
  Mux2/1 -> Bit to Integer Converter2/1
  Overwrite Values16/1 -> Mux1/4
  Overwrite Values22/1 -> Mux2/2
  Demux2/3 -> Overwrite Values23/2
  Overwrite Values7/1 -> Mux/5
  Demux1/3 -> Overwrite Values15/2
  Demux2/5 -> Overwrite Values25/2
  Overwrite Values12/1 -> Mux1/8
  Integer to Bit Converter2/1 -> Demux2/1
  Overwrite Values13/1 -> Mux1/1
  Overwrite Values4/1 -> Mux/2
  Bit to Integer Converter1/1 -> Out2/1
  Demux2/4 -> Overwrite Values24/2
  Bit to Integer Converter8/1 -> Out9/1
  Mux8/1 -> Bit to Integer Converter8/1
  Demux8/1 -> Overwrite Values2/2
  Overwrite Values81/1 -> Mux10/6
  Overwrite Values75/1 -> Mux10/8
  Overwrite Values82/1 -> Mux10/7
  Mux13/1 -> Bit to Integer Converter13/1
  Demux11/6 -> Overwrite Values89/2
  Overwrite Values86/1 -> Mux11/3
  Overwrite Values94/1 -> Mux13/1
  Demux15/1 -> Overwrite Values112/2
  Integer to Bit Converter15/1 -> Demux15/1
  Mux11/1 -> Bit to Integer Converter11/1
  Overwrite Values84/1 -> Mux11/1
  Overwrite Values83/1 -> Mux11/8
  Demux11/5 -> Overwrite Values88/2
  Demux13/8 -> Overwrite Values93/2
  Demux11/7 -> Overwrite Values90/2
  Overwrite Values88/1 -> Mux11/5
  Demux11/8 -> Overwrite Values83/2
  In14/1 -> Integer to Bit Converter11/1
  Demux11/1 -> Overwrite Values84/2
  Demux11/4 -> Overwrite Values87/2
  Integer to Bit Converter11/1 -> Demux11/1
  Overwrite Values89/1 -> Mux11/6
  Demux11/2 -> Overwrite Values85/2
  Overwrite Values118/1 -> Mux15/6
  Overwrite Values96/1 -> Mux13/2
  Overwrite Values85/1 -> Mux11/2
  Bit to Integer Converter11/1 -> Out12/1
  Overwrite Values87/1 -> Mux11/4
  Demux12/3 -> Overwrite Values121/2
  Overwrite Values119/1 -> Mux15/7
  Overwrite Values105/1 -> Mux14/3
  Overwrite Values115/1 -> Mux15/4
  Demux13/3 -> Overwrite Values97/2
  Overwrite Values104/1 -> Mux14/2
  Overwrite Values109/1 -> Mux14/6
  Demux14/4 -> Overwrite Values107/2
  Demux15/2 -> Overwrite Values113/2
  Demux14/3 -> Overwrite Values105/2
  Demux14/6 -> Overwrite Values109/2
  Demux15/3 -> Overwrite Values114/2
  Demux12/2 -> Overwrite Values120/2
  Overwrite Values92/1 -> Mux12/1
  Overwrite Values116/1 -> Mux15/5
  Overwrite Values100/1 -> Mux13/6
  Overwrite Values91/1 -> Mux12/8
  In2/1 -> Overwrite Values11/1, Overwrite Values4/1, Overwrite Values5/1, Overwrite Values6/1, Overwrite Values7/1, Overwrite Values8/1, Overwrite Values9/1, Overwrite Values10/1, Overwrite Values37/1, Overwrite Values62/1, Overwrite Values63/1, Overwrite Values64/1, Overwrite Values65/1, Overwrite Values66/1, Overwrite Values67/1, Overwrite Values36/1, Overwrite Values55/1, Overwrite Values56/1, Overwrite Values57/1, Overwrite Values58/1, Overwrite Values59/1, Overwrite Values60/1, Overwrite Values61/1, Overwrite Values54/1, Overwrite Values2/1, Overwrite Values95/1, Overwrite Values106/1, Overwrite Values117/1, Overwrite Values126/1, Overwrite Values127/1, Overwrite Values128/1, Overwrite Values1/1, Overwrite Values92/1, Overwrite Values120/1, Overwrite Values121/1, Overwrite Values122/1, Overwrite Values123/1, Overwrite Values124/1, Overwrite Values125/1, Overwrite Values91/1, Overwrite Values112/1, Overwrite Values113/1, Overwrite Values114/1, Overwrite Values115/1, Overwrite Values116/1, Overwrite Values118/1, Overwrite Values119/1, Overwrite Values111/1, Overwrite Values103/1, Overwrite Values104/1, Overwrite Values105/1, Overwrite Values107/1, Overwrite Values108/1, Overwrite Values109/1, Overwrite Values110/1, Overwrite Values102/1, Overwrite Values94/1, Overwrite Values96/1, Overwrite Values97/1, Overwrite Values98/1, Overwrite Values99/1, Overwrite Values100/1, Overwrite Values101/1, Overwrite Values93/1, Overwrite Values84/1, Overwrite Values85/1, Overwrite Values86/1, Overwrite Values87/1, Overwrite Values88/1, Overwrite Values89/1, Overwrite Values90/1, Overwrite Values83/1, Overwrite Values76/1, Overwrite Values77/1, Overwrite Values78/1, Overwrite Values79/1, Overwrite Values80/1, Overwrite Values81/1, Overwrite Values82/1, Overwrite Values75/1, Overwrite Values68/1, Overwrite Values69/1, Overwrite Values70/1, Overwrite Values71/1, Overwrite Values72/1, Overwrite Values73/1, Overwrite Values74/1, Overwrite Values3/1, Overwrite Values47/1, Overwrite Values48/1, Overwrite Values49/1, Overwrite Values50/1, Overwrite Values51/1, Overwrite Values52/1, Overwrite Values53/1, Overwrite Values46/1, Overwrite Values39/1, Overwrite Values40/1, Overwrite Values41/1, Overwrite Values42/1, Overwrite Values43/1, Overwrite Values44/1, Overwrite Values45/1, Overwrite Values38/1, Overwrite Values29/1, Overwrite Values30/1, Overwrite Values31/1, Overwrite Values32/1, Overwrite Values33/1, Overwrite Values34/1, Overwrite Values35/1, Overwrite Values28/1, Overwrite Values21/1, Overwrite Values22/1, Overwrite Values23/1, Overwrite Values24/1, Overwrite Values25/1, Overwrite Values26/1, Overwrite Values27/1, Overwrite Values20/1, Overwrite Values13/1, Overwrite Values14/1, Overwrite Values15/1, Overwrite Values16/1, Overwrite Values17/1, Overwrite Values18/1, Overwrite Values19/1, Overwrite Values12/1
  Mux15/1 -> Bit to Integer Converter15/1
  Overwrite Values120/1 -> Mux12/2
  Overwrite Values93/1 -> Mux13/8
  Overwrite Values111/1 -> Mux15/8
  In18/1 -> Integer to Bit Converter15/1
  Demux14/5 -> Overwrite Values108/2
  Demux13/1 -> Overwrite Values94/2
  Overwrite Values103/1 -> Mux14/1
  Demux12/8 -> Overwrite Values91/2
  Overwrite Values125/1 -> Mux12/7
  Demux15/4 -> Overwrite Values115/2
  Demux14/7 -> Overwrite Values110/2
  Demux13/2 -> Overwrite Values96/2
  Bit to Integer Converter14/1 -> Out15/1
  Overwrite Values101/1 -> Mux13/7
  Demux14/2 -> Overwrite Values104/2
  Demux14/1 -> Overwrite Values103/2
  Integer to Bit Converter14/1 -> Demux14/1
  In17/1 -> Integer to Bit Converter14/1
  Demux15/5 -> Overwrite Values116/2
  Overwrite Values114/1 -> Mux15/3
  Demux15/6 -> Overwrite Values118/2
  Demux15/7 -> Overwrite Values119/2
  Demux15/8 -> Overwrite Values111/2
  Mux12/1 -> Bit to Integer Converter12/1
  Overwrite Values113/1 -> Mux15/2
  Demux14/8 -> Overwrite Values102/2
  Mux14/1 -> Bit to Integer Converter14/1
  In15/1 -> Integer to Bit Converter12/1
  Overwrite Values108/1 -> Mux14/5
  Overwrite Values110/1 -> Mux14/7
  Overwrite Values107/1 -> Mux14/4
  Bit to Integer Converter15/1 -> Out16/1
  Overwrite Values124/1 -> Mux12/6
  Overwrite Values123/1 -> Mux12/5
  Overwrite Values122/1 -> Mux12/4
  Overwrite Values121/1 -> Mux12/3
  Bit to Integer Converter12/1 -> Out13/1
  Overwrite Values112/1 -> Mux15/1
  Demux12/7 -> Overwrite Values125/2
  Demux12/4 -> Overwrite Values122/2
  Demux12/6 -> Overwrite Values124/2
  Demux12/5 -> Overwrite Values123/2
  In16/1 -> Integer to Bit Converter13/1
  Integer to Bit Converter13/1 -> Demux13/1
  Demux12/1 -> Overwrite Values92/2
  Demux13/4 -> Overwrite Values98/2
  Demux13/5 -> Overwrite Values99/2
  Demux13/6 -> Overwrite Values100/2
  Demux13/7 -> Overwrite Values101/2
  Integer to Bit Converter12/1 -> Demux12/1
  Overwrite Values97/1 -> Mux13/3
  Bit to Integer Converter13/1 -> Out14/1
  Overwrite Values98/1 -> Mux13/4
  Overwrite Values102/1 -> Mux14/8
  Overwrite Values99/1 -> Mux13/5
  Demux11/3 -> Overwrite Values86/2
  Overwrite Values90/1 -> Mux11/7
  In13/1 -> Integer to Bit Converter10/1
  Demux9/1 -> Overwrite Values68/2
  Overwrite Values69/1 -> Mux9/2
  Overwrite Values73/1 -> Mux9/6
  Bit to Integer Converter10/1 -> Out11/1
  Demux10/1 -> Overwrite Values76/2
  Integer to Bit Converter9/1 -> Demux9/1
  Demux9/2 -> Overwrite Values69/2
  Demux10/6 -> Overwrite Values81/2
  Demux8/5 -> Overwrite Values126/2
  Overwrite Values117/1 -> Mux8/4
  Demux8/3 -> Overwrite Values106/2
  Demux9/8 -> Overwrite Values3/2
  Overwrite Values127/1 -> Mux8/6
  Demux8/7 -> Overwrite Values128/2
  Overwrite Values2/1 -> Mux8/1
  Demux8/6 -> Overwrite Values127/2
  Overwrite Values72/1 -> Mux9/5
  Demux8/4 -> Overwrite Values117/2
  In12/1 -> Integer to Bit Converter9/1
  Overwrite Values70/1 -> Mux9/3
  Demux8/2 -> Overwrite Values95/2
  Demux10/8 -> Overwrite Values75/2
  Overwrite Values76/1 -> Mux10/1
  Demux9/5 -> Overwrite Values72/2
  Overwrite Values78/1 -> Mux10/3
  Demux10/7 -> Overwrite Values82/2
  In7/1 -> Integer to Bit Converter8/1
  Demux9/4 -> Overwrite Values71/2
  Integer to Bit Converter8/1 -> Demux8/1
  Demux10/2 -> Overwrite Values77/2
  Demux8/8 -> Overwrite Values1/2
  Overwrite Values1/1 -> Mux8/8
  Demux9/7 -> Overwrite Values74/2
  Overwrite Values80/1 -> Mux10/5
  Overwrite Values106/1 -> Mux8/3
  Demux9/6 -> Overwrite Values73/2
  Overwrite Values74/1 -> Mux9/7
  Mux9/1 -> Bit to Integer Converter9/1
  Overwrite Values128/1 -> Mux8/7
  Overwrite Values79/1 -> Mux10/4
  Mux10/1 -> Bit to Integer Converter10/1
  Overwrite Values71/1 -> Mux9/4
  Overwrite Values77/1 -> Mux10/2
  Demux10/3 -> Overwrite Values78/2
  Overwrite Values126/1 -> Mux8/5
  Demux9/3 -> Overwrite Values70/2
  Demux10/5 -> Overwrite Values80/2
  Overwrite Values3/1 -> Mux9/8
  Integer to Bit Converter10/1 -> Demux10/1
  Overwrite Values68/1 -> Mux9/1
  Overwrite Values95/1 -> Mux8/2
  Bit to Integer Converter9/1 -> Out10/1
  Demux10/4 -> Overwrite Values79/2
